simulink model "FuzzyPD_BallBeam"  (R2016b)
settings: Solver=ode5  StartTime=0.0  StopTime=80  FixedStep=0.001  RelTol=1e-3
undefined symbols (not defined in the file or in its folder): sigbuilder_block
libraries: fuzblock x1
settings Model: Creator=HTH  LastModifiedBy=HTH

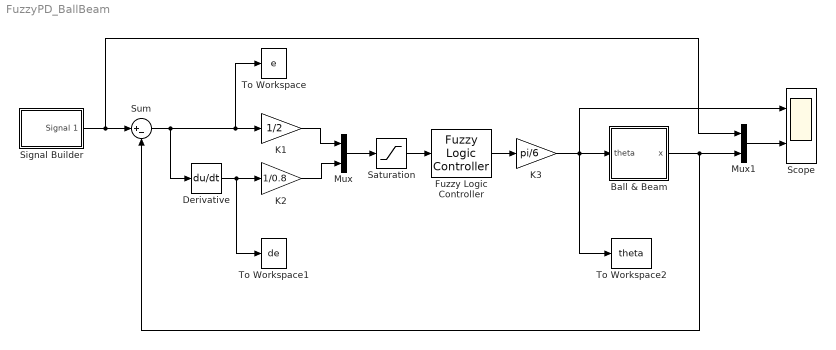
== system FuzzyPD_BallBeam ==
  Ball & Beam : Subsystem  mask{J=0.00005, R=0.02, m=0.1, b=0.01, g=9.81, x0=0, xdot0=0}
      mask prompts: J "Moment quan tinh cua bong"; R "Ban kinh bong"; m "Khoi luong bong"; b "He so ma sat"; g "Gia toc trong truong"; x0 "Vi tri dau"; xdot0 "Van toc ban dau"
  Derivative : Derivative
  Fuzzy Logic Controller : fuzblock/Fuzzy Logic  Controller  fis='FuzzyPD_BallBeam_FIS.fis'
  K1 : Gain  Gain=1/2
  K2 : Gain  Gain=1/0.8
  K3 : Gain  Gain=pi/6
  Mux : Mux  Inputs=2
  Mux1 : Mux  Inputs=2
  Saturation : Saturate  UpperLimit=1  LowerLimit=-1
  Scope : Scope  NumInputPorts=2
  Signal Builder : Subsystem  Tag=STV Subsys  LoadFcn=sigbuilder_block('load',[140.25 108 550.5 318.75 ]);  StartFcn=sigbuilder_block('start');  StopFcn=sigbuilder_block('stop');  ClipboardFcn=sigbuilder_block('clipboard');  mask(Sigbuilder block){tuvar=[0:10]}
      mask help: Simulink:masks:SigbuilderBlock_MD
      mask init:
      | if ~strcmp(get_param(bdroot(gcbh),'SimulationStatus'),'stopped') tuvar = sigbuilder_block('maskInit'); end
      settings: CopyFcn=sigbuilder_block('copy');  DeleteFcn=sigbuilder_block('delete');  ModelCloseFcn=sigbuilder_block('modelClose');  PreSaveFcn=sigbuilder_block('preSave');  PauseFcn=sigbuilder_block('pause');  ContinueFcn=sigbuilder_block('continue');  NameChangeFcn=sigbuilder_block('namechange');  OpenFcn=sigbuilder_block('open',[437.6 199.2 550.4 400 ]);  CloseFcn=sigbuilder_block('close');
      mask Display: plot(0, 0, 100, 100,[2, 2, 32, 32, 2], [68, 8, 8, 68, 68],[32, 2], [38, 38], [32, 19, 2],[53, 60, 44], [32, 17, 17, 2],[16, 16, 31, 31]);txt = getActiveGroup(gcbh);text(2, 100, txt,'verticalAlignment', 'top');
  Sum : Sum  Inputs=|+-
  To Workspace : ToWorkspace  VariableName=e  SampleTime=-1
  To Workspace1 : ToWorkspace  VariableName=de  SampleTime=-1
  To Workspace2 : ToWorkspace  VariableName=theta  SampleTime=-1
  wires:
  Fuzzy Logic Controller/1 -> K3/1
  K3/1 -> To Workspace2/1, Scope/1, Ball & Beam/1(theta)
  Mux/1 -> Saturation/1
  Ball & Beam/1(x) -> Mux1/2, Sum/2
  K1/1 -> Mux/1
  K2/1 -> Mux/2
  Saturation/1 -> Fuzzy Logic Controller/1
  Sum/1 -> Derivative/1, To Workspace/1, K1/1
  Derivative/1 -> To Workspace1/1, K2/1
  Signal Builder/1(Signal 1) -> Mux1/1, Sum/1
  Mux1/1 -> Scope/2

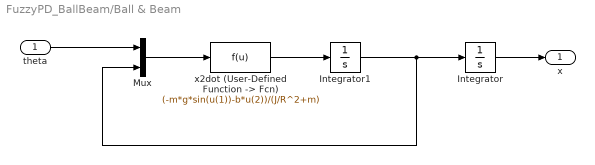
== system FuzzyPD_BallBeam/Ball & Beam ==
  theta : Inport
  Integrator : Integrator  InitialCondition=x0
  Integrator1 : Integrator  InitialCondition=xdot0
  Mux : Mux  Inputs=2
  "x2dot (User-Defined Function -> Fcn)" : Fcn  Expr=(-m*g*sin(u(1))-b*u(2))/(J/R^2+m)
  x : Outport
  wires:
  Integrator/1 -> x/1
  Integrator1/1 -> Mux/2, Integrator/1
  "x2dot (User-Defined Function -> Fcn)"/1 -> Integrator1/1
  theta/1 -> Mux/1
  Mux/1 -> "x2dot (User-Defined Function -> Fcn)"/1

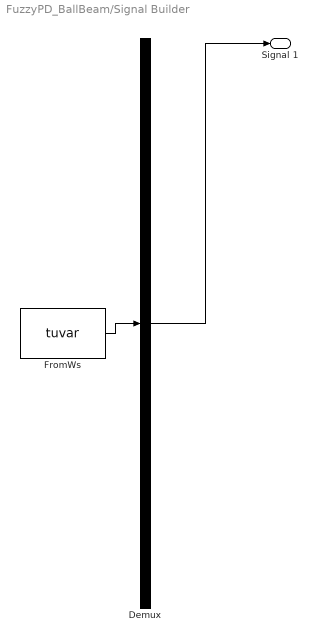
== system FuzzyPD_BallBeam/Signal Builder ==
  Demux : Demux  Tag=STV Demux  Outputs=1
  FromWs : FromWorkspace  Tag=STV FromWs  VariableName=tuvar  SampleTime=0
      SigBuilderData=|
      | common.afterFinalStr = 'Extrapolate'
      | common.sampleTime = 0
      | dataSet.timeRange = [0 80]
      | dataSet.name = 'Group 1'
      | sbobj.Groups.Name = 'Group 1'
      | sbobj.Groups.Signals.Name = 'Signal 1'
      | sbobj.Groups.Signals.XData = [0 12 12 24 24 36 36 46.5 46.5 56.8 56.8 68 68 80]
      | sbobj.Groups.Signals.YData = [0.6 0.6 -0.2 -0.2 0.96 0.96 0.41 0.41 -0.94 -0.94 -0.24 -0.24 0.58 0.58]
      | sbobj.Groups.TimeRange = [0 80]
  Signal 1 : Outport  Tag=STV Outport
  wires:
  Demux/1 -> Signal 1/1
  FromWs/1 -> Demux/1
